simulink model "cv02"  (R2024b)
settings: Solver=VariableStepAuto  StartTime=0.0  StopTime=1000  RelTol=1e-3
undefined symbols (not defined in the file): entity, m, n, ReadTime
settings Model: Creator=baron  LastModifiedBy=baron

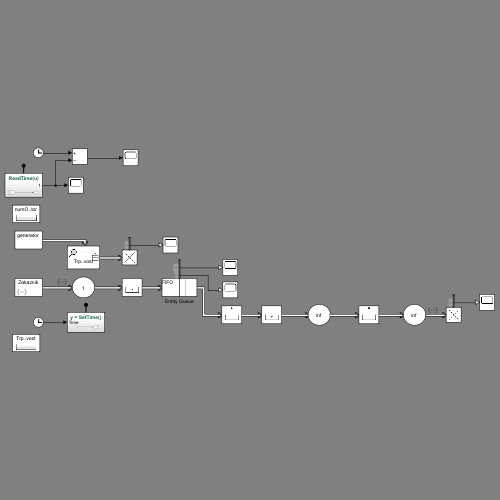
[thumbnail: Simulink's stored preview of the top-level diagram]
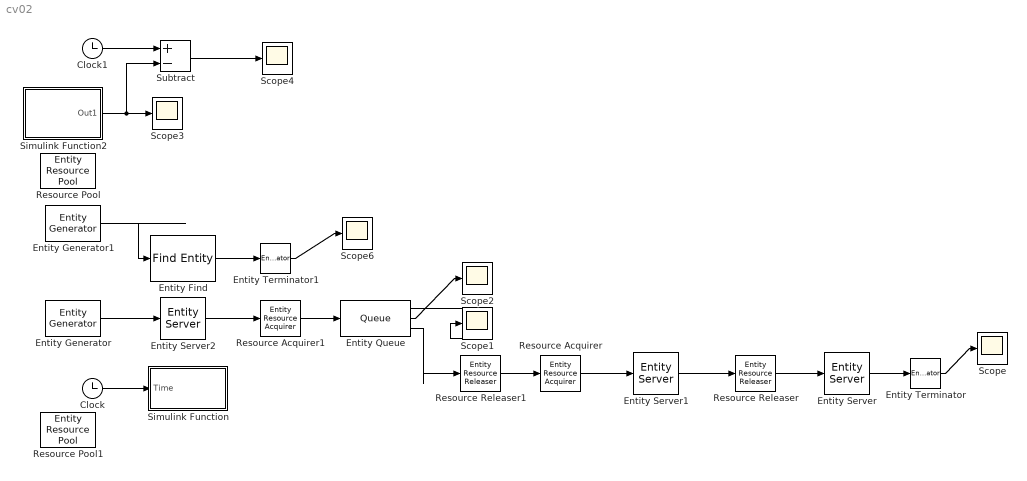
== system cv02 ==
  Clock : Clock
  Clock1 : Clock
  Entity Find : FindEntity  InputPortMessageModes=m  OutputPortMessageModes=m  ResourceName=Trpelivost  EnableOutput=on  EntityFilter=on  MatchingCondition=|
      | % match = isequal(trigger.Attribute1, entity.Attribute1);
      | 
      | now = SetTime()
      | 
      | match = (now-entity.timeStart)>entity.Trpelivost;
      settings: OutputPortMap=o6
  Entity Generator : EntityGenerator  OutputPortMessageModes=m  TimeSource=MATLAB action  IntergenerationTimeAction=|  GenerateAction=|  AttributeName=timeStart|timeEnd|timeCall|Trpelivost  AttributeInitialValue=1|1|1|3  EntityType=Structured  EntityTypeName=Zakaznik
      IntergenerationTimeAction=|
      | dt = rand(1,1);
      | persistent rngInit;
      | if isempty(rngInit)
      |     seed = 12345;
      |     rng(seed);
      |     rngInit = true;
      | end
      | 
      | % Pattern: Uniform distribution
      | % m: Minimum, M: Maximum
      | m = 0.1; M = 5;
      | dt = m + (M - m) * rand;
      GenerateAction=|
      | persistent rngInit;
      | if isempty(rngInit)
      |     seed = 12345;
      |     rng(seed);
      |     rngInit = true;
      | end
      | 
      | % Pattern: Uniform distribution
      | % m: Minimum, M: Maximum
      | m = 5; M = 15;
      | entity.timeCall = m + (M - m) * rand;
  Entity Generator1 : EntityGenerator  OutputPortMessageModes=m  Period=0.01  EntityType=Structured  EntityTypeName=generator
  Entity Queue : Queue  InputPortMessageModes=m  OutputPortMessageModes=n,n,m  Capacity=inf  NumberEntitiesInBlock=on  AverageWait=on
      settings: OutputPortMap=o1,o2,o5
  Entity Server : EntityServer  InputPortMessageModes=m  OutputPortMessageModes=m  Capacity=inf  ExitAction=ReadTime(entity.timeStart)
  Entity Server1 : EntityServer  InputPortMessageModes=m  OutputPortMessageModes=m  Capacity=inf  ServiceTimeSource=Attribute  ServiceTimeAttributeName=timeCall
  Entity Server2 : EntityServer  InputPortMessageModes=m  OutputPortMessageModes=m  Capacity=1  ServiceTimeValue=0  EntryAction=entity.timeStart = SetTime()
  Entity Terminator : EntityTerminator  InputPortMessageModes=m  NumberEntitiesArrived=on
      settings: OutputPortMap=o0
  Entity Terminator1 : EntityTerminator  InputPortMessageModes=m  NumberEntitiesArrived=on
      settings: OutputPortMap=o0
  Resource Acquirer : EntityResourceAcquirer  InputPortMessageModes=m  OutputPortMessageModes=m  ResourceName=numOfOperator
      settings: OutputPortMap=o3
  Resource Acquirer1 : EntityResourceAcquirer  InputPortMessageModes=m  OutputPortMessageModes=m  ResourceName=Trpelivost
      settings: OutputPortMap=o3
  Resource Releaser : EntityResourceReleaser  InputPortMessageModes=m  OutputPortMessageModes=m  ResourceToRelease=Selected  ResourceName=numOfOperator  ResourceAmount=1
  Resource Releaser1 : EntityResourceReleaser  InputPortMessageModes=m  OutputPortMessageModes=m  ResourceToRelease=Selected  ResourceName=Trpelivost  ResourceAmount=1
  Resource Pool : EntityResourcePool  ResourceName=numOfOperator  ResourceAmount=3
  Resource Pool1 : EntityResourcePool  ResourceName=Trpelivost  ResourceAmount=1000
  Scope{,1..4,6} (6 alike) : Scope
  Simulink Function : Subsystem  TreatAsAtomicUnit=on
  Simulink Function2 : Subsystem  TreatAsAtomicUnit=on
  Subtract : Sum  Inputs=+-
  wires:
  Entity Generator/1 -> Entity Server2/1
  Clock1/1 -> Subtract/1
  Subtract/1 -> Scope4/1
  Simulink Function2/1(Out1) -> Scope3/1, Subtract/2
  Entity Generator1/1 -> Entity Find/1
  Entity Find/1 -> Entity Terminator1/1
  Clock/1 -> Simulink Function/1(Time)
  Entity Server2/1 -> Resource Acquirer1/1
  Entity Terminator1/1 -> Scope6/1
  Resource Acquirer1/1 -> Entity Queue/1
  Entity Queue/2 -> Scope2/1
  Entity Queue/1 -> Scope1/1
  Entity Queue/3 -> Resource Releaser1/1
  Resource Releaser1/1 -> Resource Acquirer/1
  Resource Acquirer/1 -> Entity Server1/1
  Entity Server1/1 -> Resource Releaser/1
  Resource Releaser/1 -> Entity Server/1
  Entity Terminator/1 -> Scope/1
  Entity Server/1 -> Entity Terminator/1

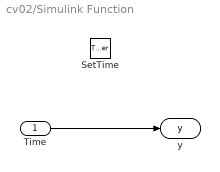
== system cv02/Simulink Function ==
  Time : Inport
  SetTime : TriggerPort  TriggerType=function-call  IsSimulinkFunction=on  FunctionName=SetTime  FunctionVisibility=scoped  VariantControl=(inherit)
  y : ArgOut  DisableCoverage=on  ArgumentName=y
  wires:
  Time/1 -> y/1

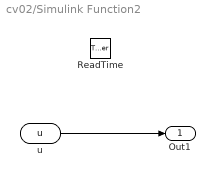
== system cv02/Simulink Function2 ==
  ReadTime : TriggerPort  TriggerType=function-call  IsSimulinkFunction=on  FunctionName=ReadTime  FunctionVisibility=scoped  VariantControl=(inherit)
  u : ArgIn  DisableCoverage=on  ArgumentName=u
  Out1 : Outport
  wires:
  u/1 -> Out1/1
